simulink model "Feedforward_antiwindup_sim"  (R2020b)
settings: Solver=ode45  StartTime=0.0  StopTime=5  RelTol=1e-3
undefined symbols (not defined in the file or in its folder): BEMF_comp, Beq_hat, ctrl, daq, degs2rpm, denHwa, denHws, drv, friction_comp, gbox, inertia_comp, Jeq_hat, mot, numHwa, numHws, rads2rpm, rpm2rads, sens, tau_hat
libraries: simulink x1
settings Model: Creator=gioel  LastModifiedBy=giuli
settings DataIOCC: ReturnWorkspaceOutputs=off

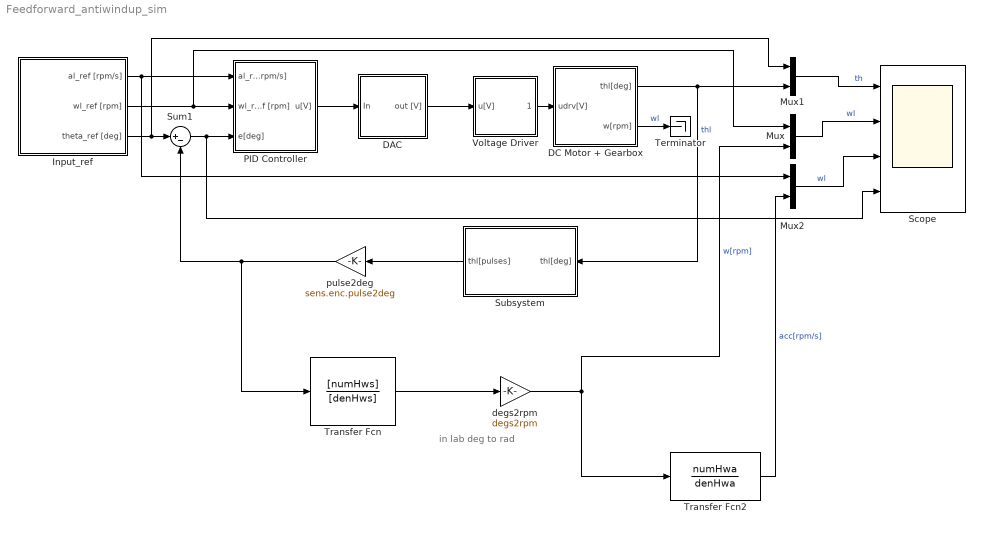
== system Feedforward_antiwindup_sim ==
  note: in lab deg to rad
  DAC : Subsystem
  DC Motor + Gearbox : Subsystem
  Input_ref : Subsystem
  Mux : Mux  Inputs=2
  Mux1 : Mux  Inputs=2
  Mux2 : Mux  Inputs=2
  PID Controller : Subsystem
  Scope : Scope  NumInputPorts=4
  Subsystem : Subsystem
  Sum1 : Sum  Inputs=|+-
  Terminator : Terminator
  Transfer Fcn : TransferFcn  Numerator=[numHws]  Denominator=[denHws]
  Transfer Fcn2 : TransferFcn  Numerator=numHwa  Denominator=denHwa
  Voltage Driver : Subsystem
  degs2rpm : Gain  Gain=degs2rpm
  pulse2deg : Gain  Gain=sens.enc.pulse2deg
  wires:
  PID Controller/1(u[V]) -> DAC/1(In)
  pulse2deg/1 -> Transfer Fcn/1, Sum1/2
  DAC/1(out [V]) -> Voltage Driver/1(u[V])
  Subsystem/1(thl[pulses]) -> pulse2deg/1
  Voltage Driver/1(udrv[V]) -> DC Motor + Gearbox/1(udrv[V])
  DC Motor + Gearbox/1(thl[deg]) -> Mux1/2, Subsystem/1(thl[deg])  "thl"
  Input_ref/3(theta_ref [deg]) -> Mux1/1, Sum1/1
  Sum1/1 -> Scope/4, PID Controller/3(e[deg])
  Input_ref/2(wl_ref [rpm]) -> Mux/1, PID Controller/2("wl_ref [rpm] ")
  Input_ref/1(al_ref [rpm/s]) -> Mux2/1, PID Controller/1("al_ref [rpm/s]  ")
  degs2rpm/1 -> Transfer Fcn2/1, Mux/2  "w[rpm]"
  Transfer Fcn/1 -> degs2rpm/1
  Mux/1 -> Scope/2  "wl"
  Mux1/1 -> Scope/1  "th"
  Transfer Fcn2/1 -> Mux2/2  "acc[rpm/s]"
  Mux2/1 -> Scope/3  "wl"
  DC Motor + Gearbox/2(w[rpm]) -> Terminator/1  "wl"

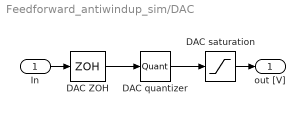
== system Feedforward_antiwindup_sim/DAC ==
  In : Inport
  DAC quantizer : Quantizer  QuantizationInterval=daq.dac.q
  DAC saturation : Saturate  UpperLimit=daq.dac.fs  LowerLimit=-daq.dac.fs
  DAC ZOH : ZeroOrderHold  SampleTime=0.001
  out [V] : Outport
  wires:
  DAC ZOH/1 -> DAC quantizer/1
  DAC quantizer/1 -> DAC saturation/1
  In/1 -> DAC ZOH/1
  DAC saturation/1 -> out [V]/1

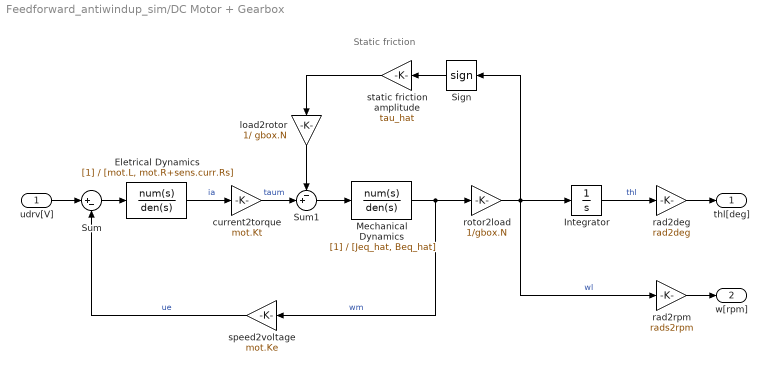
== system Feedforward_antiwindup_sim/DC Motor + Gearbox ==
  note: Static friction
  udrv[V] : Inport
  Eletrical Dynamics : TransferFcn  Denominator=[mot.L, mot.R+sens.curr.Rs]
  Integrator : Integrator
  Mechanical Dynamics : TransferFcn  Denominator=[Jeq_hat, Beq_hat]
  Sign : Signum  ZeroCross=off
  Sum : Sum  Inputs=|+-
  Sum1 : Sum  Inputs=-+|
  current2torque : Gain  Gain=mot.Kt
  load2rotor : Gain  Gain=1/ gbox.N
  rad2deg : Gain  Gain=rad2deg
  "rad2rpm " : Gain  Gain=rads2rpm
  rotor2load : Gain  Gain=1/gbox.N
  speed2voltage : Gain  Gain=mot.Ke
  static friction amplitude : Gain  Gain=tau_hat
  thl[deg] : Outport  VectorParamsAs1DForOutWhenUnconnected=off
  w[rpm] : Outport  Port=2  VectorParamsAs1DForOutWhenUnconnected=off
  wires:
  Eletrical Dynamics/1 -> current2torque/1  "ia"
  udrv[V]/1 -> Sum/1
  Sum/1 -> Eletrical Dynamics/1
  current2torque/1 -> Sum1/2  "taum"
  Sum1/1 -> Mechanical Dynamics/1
  Mechanical Dynamics/1 -> rotor2load/1, speed2voltage/1  "wm"
  rotor2load/1 -> Integrator/1, "rad2rpm "/1, Sign/1  "wl"
  Integrator/1 -> rad2deg/1  "thl"
  rad2deg/1 -> thl[deg]/1
  "rad2rpm "/1 -> w[rpm]/1
  static friction amplitude/1 -> load2rotor/1
  Sign/1 -> static friction amplitude/1
  speed2voltage/1 -> Sum/2  "ue"
  load2rotor/1 -> Sum1/1

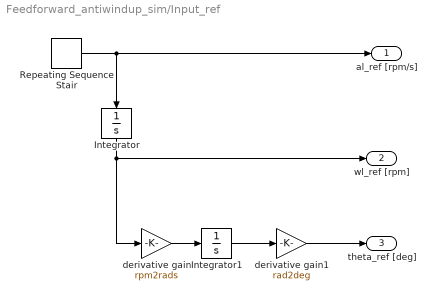
== system Feedforward_antiwindup_sim/Input_ref ==
  Integrator : Integrator
  Integrator1 : Integrator
  Repeating Sequence Stair : simulink/Sources/Repeating Sequence Stair  OutValues=[900 0 -900 -900 0 900].'  tsamp=0.5  OutMin=[]  OutMax=[]  OutDataTypeStr=double  OutputDataTypeScalingMode=double  OutDataType=fixdt(0,8)  ConRadixGroup=Best Precision: Vector-wise  OutScaling=2^-12
  derivative gain : Gain  Gain=rpm2rads
  derivative gain1 : Gain  Gain=rad2deg
  al_ref [rpm/s] : Outport  VectorParamsAs1DForOutWhenUnconnected=off
  wl_ref [rpm] : Outport  Port=2  VectorParamsAs1DForOutWhenUnconnected=off
  theta_ref [deg] : Outport  Port=3  VectorParamsAs1DForOutWhenUnconnected=off
  wires:
  Repeating Sequence Stair/1 -> al_ref [rpm/s]/1, Integrator/1
  Integrator1/1 -> derivative gain1/1
  derivative gain1/1 -> theta_ref [deg]/1
  derivative gain/1 -> Integrator1/1
  Integrator/1 -> wl_ref [rpm]/1, derivative gain/1

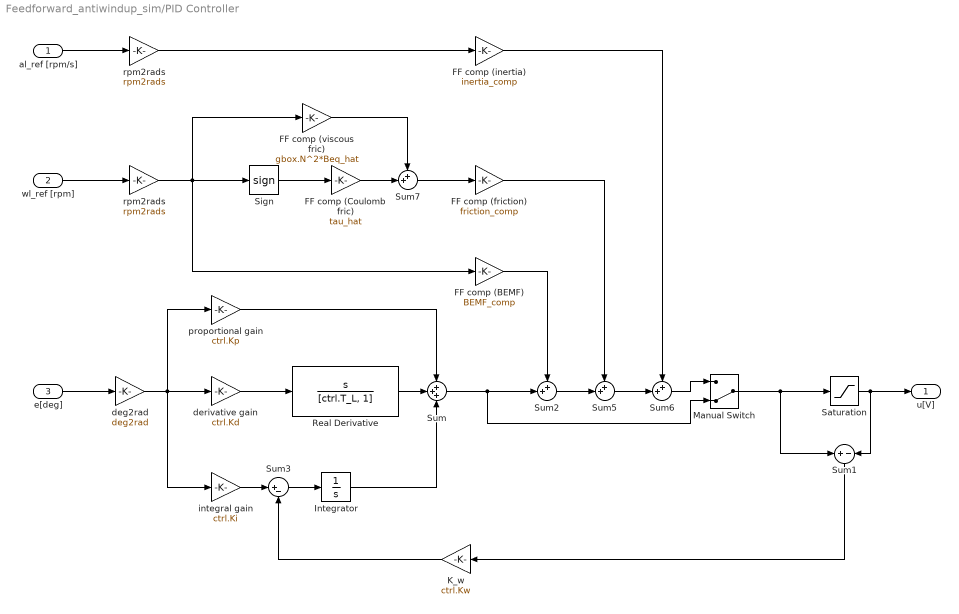
== system Feedforward_antiwindup_sim/PID Controller ==
  "al_ref [rpm/s]  " : Inport
  "wl_ref [rpm] " : Inport  Port=2
  e[deg] : Inport  Port=3
  FF comp (Coulomb fric) : Gain  Gain=tau_hat
  FF comp (viscous fric) : Gain  Gain=gbox.N^2*Beq_hat
  FF comp (BEMF) : Gain  Gain=BEMF_comp
  FF comp (friction) : Gain  Gain=friction_comp
  FF comp (inertia) : Gain  Gain=inertia_comp
  Integrator : Integrator
  K_w : Gain  Gain=ctrl.Kw
  Manual Switch : ManualSwitch  CurrentSetting=0
  Real Derivative : TransferFcn  Numerator=[1 0]  Denominator=[ctrl.T_L, 1]
  Saturation : Saturate  UpperLimit=10  LowerLimit=-10
  "Sign " : Signum  ZeroCross=off
  Sum : Sum  Inputs=+++
  Sum1 : Sum  Inputs=+|-
  Sum{2,5..7} (4 alike) : Sum  Inputs=++|
  Sum3 : Sum  Inputs=|+-
  deg2rad : Gain  Gain=deg2rad
  derivative gain : Gain  Gain=ctrl.Kd
  integral gain : Gain  Gain=ctrl.Ki
  proportional gain : Gain  Gain=ctrl.Kp
  rpm2rads : Gain  Gain=rpm2rads
  "rpm2rads " : Gain  Gain=rpm2rads
  u[V] : Outport
  wires:
  Saturation/1 -> Sum1/2, u[V]/1
  Real Derivative/1 -> Sum/2
  proportional gain/1 -> Sum/1
  Sum1/1 -> K_w/1
  derivative gain/1 -> Real Derivative/1
  deg2rad/1 -> integral gain/1, derivative gain/1, proportional gain/1
  Integrator/1 -> Sum/3
  integral gain/1 -> Sum3/1
  Sum3/1 -> Integrator/1
  K_w/1 -> Sum3/2
  Sum5/1 -> Sum6/2
  Sum7/1 -> FF comp (friction)/1
  Sum2/1 -> Sum5/2
  FF comp (Coulomb fric)/1 -> Sum7/2
  FF comp (viscous fric)/1 -> Sum7/1
  rpm2rads/1 -> FF comp (inertia)/1
  "Sign "/1 -> FF comp (Coulomb fric)/1
  "rpm2rads "/1 -> FF comp (BEMF)/1, FF comp (viscous fric)/1, "Sign "/1
  Sum/1 -> Manual Switch/2, Sum2/2
  "al_ref [rpm/s]  "/1 -> rpm2rads/1
  e[deg]/1 -> deg2rad/1
  "wl_ref [rpm] "/1 -> "rpm2rads "/1
  FF comp (BEMF)/1 -> Sum2/1
  FF comp (friction)/1 -> Sum5/1
  FF comp (inertia)/1 -> Sum6/1
  Sum6/1 -> Manual Switch/1
  Manual Switch/1 -> Sum1/1, Saturation/1

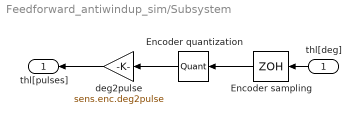
== system Feedforward_antiwindup_sim/Subsystem ==
  thl[deg] : Inport
  Encoder quantization : Quantizer  QuantizationInterval=sens.enc.pulse2deg
  Encoder sampling : ZeroOrderHold  SampleTime=-1
  deg2pulse : Gain  Gain=sens.enc.deg2pulse
  thl[pulses] : Outport
  wires:
  thl[deg]/1 -> Encoder sampling/1
  Encoder quantization/1 -> deg2pulse/1
  Encoder sampling/1 -> Encoder quantization/1
  deg2pulse/1 -> thl[pulses]/1

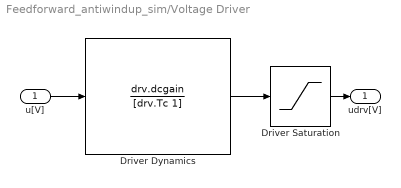
== system Feedforward_antiwindup_sim/Voltage Driver ==
  u[V] : Inport
  Driver Dynamics : TransferFcn  Numerator=drv.dcgain  Denominator=[drv.Tc 1]
  Driver Saturation : Saturate  UpperLimit=12  LowerLimit=-12
  udrv[V] : Outport
  wires:
  Driver Dynamics/1 -> Driver Saturation/1
  Driver Saturation/1 -> udrv[V]/1
  u[V]/1 -> Driver Dynamics/1
